simulink model "sim1_"  (R2024b)
settings: Solver=VariableStepAuto  StartTime=0.0  StopTime=200  RelTol=1e-3
settings Model: Creator=callm  LastModifiedBy=callm

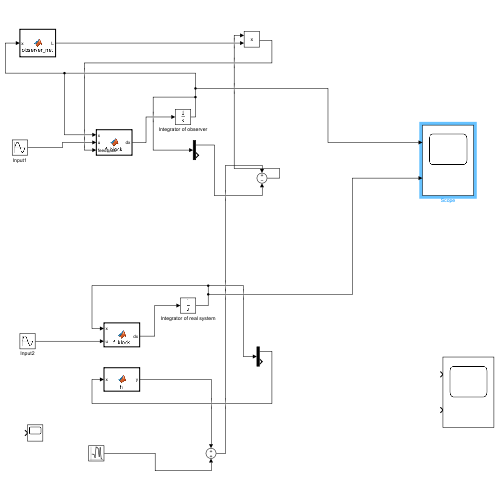
[thumbnail: Simulink's stored preview of the top-level diagram]
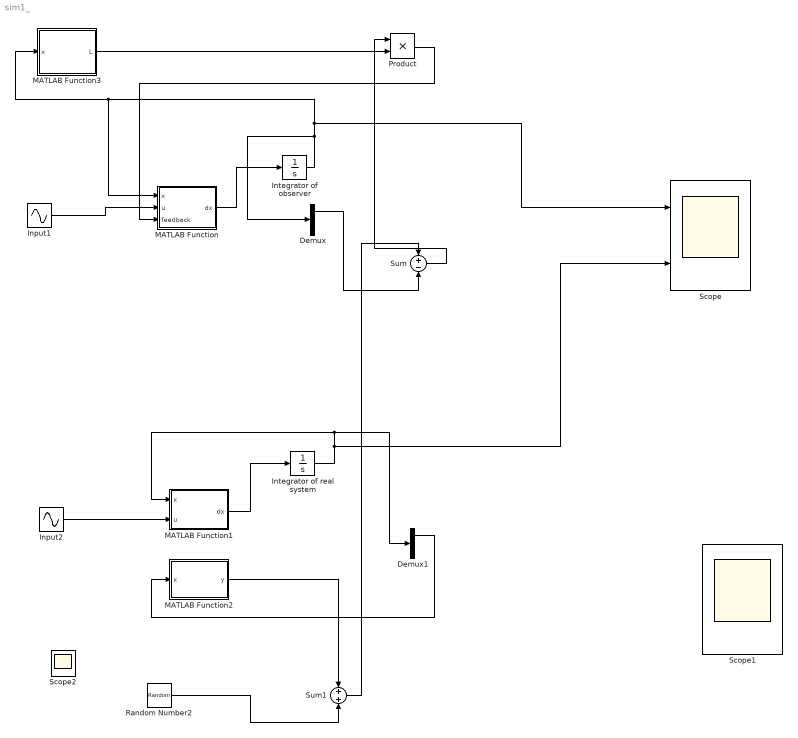
== system sim1_ ==
  Demux : Demux  Outputs=2
  Demux1 : Demux  Outputs=2
  Input1 : Sin  Amplitude=0.37  Frequency=1.2  Phase=pi/2  SampleTime=0
  Input2 : Sin  Amplitude=0.37  Frequency=1.2  Phase=pi/2  SampleTime=0
  Integrator of observer : Integrator  InitialCondition=[0;0]
  Integrator of real system : Integrator  InitialCondition=[1;1]
  MATLAB Function : MATLAB Function  TreatAsAtomicUnit=on
  MATLAB Function1 : MATLAB Function  TreatAsAtomicUnit=on
  MATLAB Function2 : MATLAB Function  TreatAsAtomicUnit=on
  MATLAB Function3 : MATLAB Function  TreatAsAtomicUnit=on
  Product : Product
  Random Number2 : RandomNumber  Variance=0.005  SampleTime=0.1
  Scope : Scope  NumInputPorts=2
  Scope1 : Scope  NumInputPorts=2
  Scope2 : Scope
  Sum : Sum  Inputs=+-
  Sum1 : Sum
  wires:
  MATLAB Function/1(dx) -> Integrator of observer/1
  Input2/1 -> MATLAB Function1/2(u)
  MATLAB Function1/1(dx) -> Integrator of real system/1
  Integrator of real system/1 -> Scope/2, MATLAB Function1/1(x), Demux1/1
  Input1/1 -> MATLAB Function/2(u)
  Demux/1 -> Sum/2
  Integrator of observer/1 -> Demux/1, Scope/1, MATLAB Function/1(x), MATLAB Function3/1(x)
  Product/1 -> MATLAB Function/3(feedback)
  Demux1/1 -> MATLAB Function2/1(x)
  MATLAB Function3/1(L) -> Product/2
  Sum/1 -> Product/1
  Random Number2/1 -> Sum1/2
  MATLAB Function2/1(y) -> Sum1/1
  Sum1/1 -> Sum/1

== matlab function sim1_/MATLAB Function ==
  data: x input; dx output; u input; feedback input
function dx = f_block(x, u, feedback)
 
%#codegen

% 明确指定维度
assert(isa(x, 'double'));
assert(isa(u, 'double'));
assert(all(size(x) == [2, 1]));

% 明确输出维度
dx = zeros(2, 1);

% Duffing 方程参数
alpha = -1;
beta = 1;
delta = 0.3;

x1 = x(1);
x2 = x(2);

dx(1) = x2;
dx(2) = u - delta*x2 - alpha*x1 - beta*x1^3;

dx=dx+feedback;

end

== matlab function sim1_/MATLAB Function3 ==
  data: x input size=[2 1]; L output size=[2 1]
function L = observer_net(x)
%#codegen

% 明确指定输出维度
L = zeros(2, 1);

x1 = x(1);
x2 = x(2);

persistent F11_grid F12_grid F22_grid
if isempty(F11_grid)
    data = coder.load('P_gridded_interpolants.mat');
    F11_grid = data.F11_grid;
    F12_grid = data.F12_grid;
    F22_grid = data.F22_grid;
end

p11 = F11_grid(x1, x2);
p12 = F12_grid(x1, x2);
p22 = F22_grid(x1, x2);

P = [p11, p12; p12, p22];


L = 2.5* (P \ [1;0]);

end

== matlab function sim1_/MATLAB Function1 ==
  data: x input; dx output; u input
function dx = f_block(x, u)
%#codegen

% 明确指定维度
assert(isa(x, 'double'));
assert(isa(u, 'double'));
assert(all(size(x) == [2, 1]));

% 明确输出维度
dx = zeros(2, 1);

% Duffing 方程参数
alpha = -1;
beta = 1;
delta = 0.3;

x1 = x(1);
x2 = x(2);

dx(1) = x2;
dx(2) = u - delta*x2 - alpha*x1 - beta*x1^3;

end

== matlab function sim1_/MATLAB Function2 ==
  data: x input; y output size=[1,1]
function y = h(x)

y = x(1);

end
